simulink model "fourBusCase1"  (R2018b)
settings: Solver=FixedStepAuto  StartTime=0  StopTime=5  FixedStep=Ts  RelTol=1e-3
StartFcn:
  | clear
  | UserData = '4bus_case1.xlsx';
  | SimplusGT.Toolbox.Main();
undefined symbols (not defined in the file): ApparatusDiscreDamping, ApparatusPara, ApparatusPowerFlow, ApparatusType, OtherInputs, Ts, Wbase, x_e, Ybase, Zbase
libraries: powerlib x16, SimplusGT x7
settings Model: Creator=y_zhu  LastModifiedBy=y_zhu

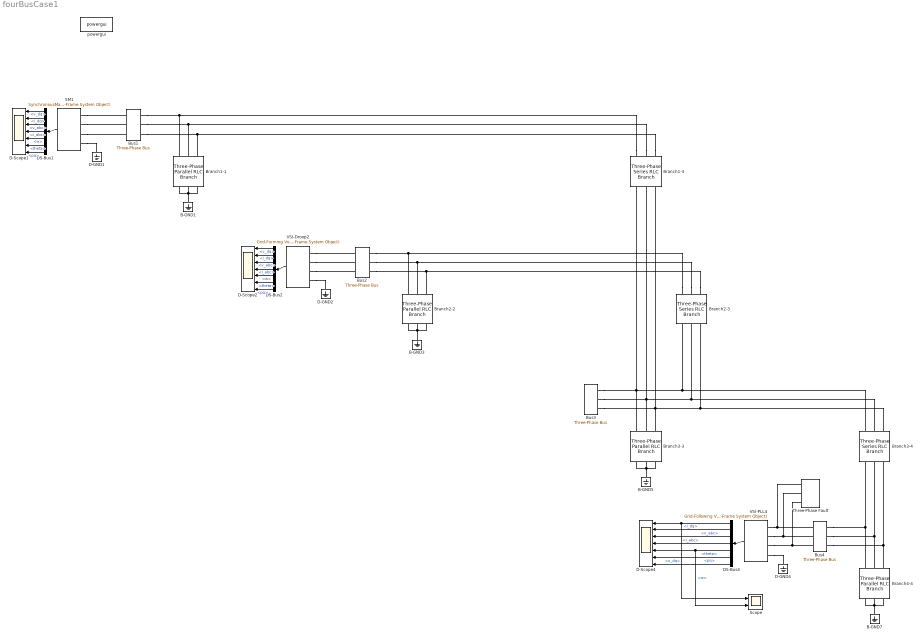
== system fourBusCase1 ==
  B-GND{1,3,5,7} (4 alike) : powerlib/Elements/Ground  LConnTagsString=a
  Branch1-1 : powerlib/Elements/Three-Phase Parallel RLC Branch  LConnTagsString=A|B|C  RConnTagsString=A|B|C  BranchType=RC  Resistance=(0.16534)*Zbase  Inductance=(Inf)*Zbase/Wbase  Capacitance=(0.238)*Ybase/Wbase  Measurements=None
      settings: SourceProductName=Simscape Power Systems  SourceProductBaseCode=PS
  Branch1-3 : powerlib/Elements/Three-Phase Series RLC Branch  LConnTagsString=A|B|C  RConnTagsString=A|B|C  BranchType=RL  Resistance=(0.004)*Zbase  Inductance=(0.057)*Zbase/Wbase  Capacitance=1e-6  Measurements=None
  Branch2-2 : powerlib/Elements/Three-Phase Parallel RLC Branch  LConnTagsString=A|B|C  RConnTagsString=A|B|C  BranchType=RLC  Resistance=(15.9719)*Zbase  Inductance=(41.1523)*Zbase/Wbase  Capacitance=(0.0368)*Ybase/Wbase  Measurements=None
      settings: SourceProductName=Simscape Power Systems  SourceProductBaseCode=PS
  Branch2-3 : powerlib/Elements/Three-Phase Series RLC Branch  LConnTagsString=A|B|C  RConnTagsString=A|B|C  BranchType=RL  Resistance=(0.0029)*Zbase  Inductance=(0.0734)*Zbase/Wbase  Capacitance=1e-6  Measurements=None
  Branch3-3 : powerlib/Elements/Three-Phase Parallel RLC Branch  LConnTagsString=A|B|C  RConnTagsString=A|B|C  BranchType=RLC  Resistance=(12.2146)*Zbase  Inductance=(12.216)*Zbase/Wbase  Capacitance=(2.142)*Ybase/Wbase  Measurements=None
      settings: SourceProductName=Simscape Power Systems  SourceProductBaseCode=PS
  Branch3-4 : powerlib/Elements/Three-Phase Series RLC Branch  LConnTagsString=A|B|C  RConnTagsString=A|B|C  BranchType=L  Resistance=(0)*Zbase  Inductance=(0.039)*Zbase/Wbase  Capacitance=1e-6  Measurements=None
  Branch4-4 : powerlib/Elements/Three-Phase Parallel RLC Branch  LConnTagsString=A|B|C  RConnTagsString=A|B|C  BranchType=RC  Resistance=(0.25293)*Zbase  Inductance=(Inf)*Zbase/Wbase  Capacitance=(0.95725)*Ybase/Wbase  Measurements=None
      settings: SourceProductName=Simscape Power Systems  SourceProductBaseCode=PS
  Bus{1..4} (4 alike) : SimplusGT/Three-Phase Bus  Vbase=1  Sbase=1
      settings: SourceProductName=Simplus Grid Tool
  D-GND1 : powerlib/Elements/Ground  LConnTagsString=a
  D-GND2 : powerlib/Elements/Ground  LConnTagsString=a
  D-GND4 : powerlib/Elements/Ground  LConnTagsString=a
  D-Scope1 : Scope  NumInputPorts=7
  D-Scope2 : Scope  NumInputPorts=7
  D-Scope4 : Scope  NumInputPorts=7
  DS-Bus1 : BusSelector  OutputSignals=v_dq,i_dq,v_abc,i_abc,w,theta,pq
  DS-Bus2 : BusSelector  OutputSignals=v_dq,i_dq,v_abc,i_abc,w,theta,pq
  DS-Bus4 : BusSelector  OutputSignals=v_dq,i_dq,v_abc,i_abc,w,theta,pq
  SM1 : SimplusGT/SynchronousMachineFull_Cyp_SMAVRPSSGOV (dq-Frame System Object)  Ts=Ts  Sbase=Sbase  Vbase=Vbase  Wbase=Wbase  ApparatusType=ApparatusType{1}  ApparatusPara=ApparatusPara{1}  PowerFlow=ApparatusPowerFlow{1}  x0=x_e{1}  OtherInputs=OtherInputs{1}  DiscreMethod=Hybrid Trapezoidal  EnableInsideModification=off  DiscreDampingFlag=on  DiscreDampingValue=ApparatusDiscreDamping{1}  LinearizationTimes=1  DirectFeedthrough=off
      settings: SourceProductName=Simplus Grid Tool
  Scope : Scope  NumInputPorts=2
  Three-Phase Fault : powerlib/Elements/Three-Phase Fault  InitialStates=0  FaultA=on  FaultB=on  FaultC=on  GroundFault=on  SwitchTimes="[2+1/60  2+3/60]"  External=off  SwitchStatus=NaN  FaultResistance=0.001  GroundResistance=0.01  SnubberResistance=1e6  SnubberCapacitance=inf  Measurements=None
  VSI-Droop2 : SimplusGT/Grid-Forming Voltage-Source Inverter (dq-Frame System Object)  Ts=Ts  Sbase=Sbase  Vbase=Vbase  Wbase=Wbase  ApparatusType=ApparatusType{2}  ApparatusPara=ApparatusPara{2}  PowerFlow=ApparatusPowerFlow{2}  x0=x_e{2}  OtherInputs=OtherInputs{2}  DiscreMethod=Hybrid Trapezoidal  EnableInsideModification=off  DiscreDampingFlag=on  DiscreDampingValue=ApparatusDiscreDamping{2}  LinearizationTimes=1  DirectFeedthrough=off
      settings: SourceProductName=Simplus Grid Tool
  VSI-PLL4 : SimplusGT/Grid-Following Voltage-Source Inverter (dq-Frame System Object)  Ts=Ts  Sbase=Sbase  Vbase=Vbase  Wbase=Wbase  ApparatusType=ApparatusType{4}  ApparatusPara=ApparatusPara{4}  PowerFlow=ApparatusPowerFlow{4}  x0=x_e{4}  OtherInputs=OtherInputs{4}  DiscreMethod=Hybrid Trapezoidal  EnableInsideModification=off  DiscreDampingFlag=on  DiscreDampingValue=ApparatusDiscreDamping{4}  LinearizationTimes=1  DirectFeedthrough=off
      settings: SourceProductName=Simplus Grid Tool
  powergui : powerlib/powergui  Priority=1  SimulationMode=Discrete  SampleTime=Ts  frequency=60  Iterations=50  frequencyindice=0  Pbase=100e6  ErrMax=1e-4  UnitsV=kV  UnitsW=MW  buscounter=0  FunctionMessages=off  echomessages=off  EnableUseOfTLC=off  CurrentSourceSwitches=off  DisableSnubberDevices=off  DisableRonSwitches=off  DisableVfSwitches=off  DisplayEquations=off  SolverType=Tustin/Backward Euler (TBE)  Interpol=off  ExternalGateDelay=off  methode=off  Ts=100  x0status=blocks  SPID=off  SwTol=0  HookPort=off  RestoreLinks=warning  ResistiveCurrentMeasurement=off  Frange=[0:2:500]  Ylog=off  Xlog=on  ShowGrid=off  save=off  variable=ZData  structure=0  ZoomFFT=off  StartTime=0.0  cycles=1  DisplayStyle=1  fundamental=60  FreqAxis=off  MaxFrequency=1000  frequencyindicesteady=1  RmsSteady=1  display=off
  wires:
  SM1/1 -> DS-Bus1/1
  DS-Bus1/1 -> D-Scope1/1  "<v_dq>"
  DS-Bus1/2 -> D-Scope1/2  "<i_dq>"
  DS-Bus1/3 -> D-Scope1/3  "<v_abc>"
  DS-Bus1/4 -> D-Scope1/4  "<i_abc>"
  DS-Bus1/5 -> D-Scope1/5  "<w>"
  DS-Bus1/6 -> D-Scope1/6  "<theta>"
  DS-Bus1/7 -> D-Scope1/7  "<pq>"
  VSI-Droop2/1 -> DS-Bus2/1
  DS-Bus2/1 -> D-Scope2/1  "<v_dq>"
  DS-Bus2/2 -> D-Scope2/2  "<i_dq>"
  DS-Bus2/3 -> D-Scope2/3  "<v_abc>"
  DS-Bus2/4 -> D-Scope2/4  "<i_abc>"
  DS-Bus2/5 -> D-Scope2/5  "<w>"
  DS-Bus2/6 -> D-Scope2/6  "<theta>"
  DS-Bus2/7 -> D-Scope2/7  "<pq>"
  VSI-PLL4/1 -> DS-Bus4/1
  DS-Bus4/2 -> D-Scope4/2  "<i_dq>"
  DS-Bus4/3 -> D-Scope4/3  "<v_abc>"
  DS-Bus4/5 -> Scope/2, D-Scope4/5  "<w>"
  DS-Bus4/6 -> D-Scope4/6  "<theta>"
  DS-Bus4/7 -> D-Scope4/7  "<pq>"
  DS-Bus4/1 -> Scope/1, D-Scope4/1  "<v_dq>"
  DS-Bus4/4 -> D-Scope4/4  "<i_abc>"
  connections:
  SM1/LConn4 -- D-GND1/LConn1
  VSI-Droop2/LConn4 -- D-GND2/LConn1
  VSI-PLL4/LConn4 -- D-GND4/LConn1
  Branch1-1/RConn1 -- Branch1-1/RConn2 -- Branch1-1/RConn3 -- B-GND1/LConn1
  Branch2-2/RConn1 -- Branch2-2/RConn2 -- Branch2-2/RConn3 -- B-GND3/LConn1
  Branch3-3/RConn1 -- Branch3-3/RConn2 -- Branch3-3/RConn3 -- B-GND5/LConn1
  Branch4-4/RConn1 -- Branch4-4/RConn2 -- Branch4-4/RConn3 -- B-GND7/LConn1
  Branch1-3/RConn1 -- Bus3/RConn1 -- Branch3-3/LConn1 -- Branch3-4/LConn1 -- Branch2-3/RConn1
  Branch1-3/RConn2 -- Bus3/RConn2 -- Branch3-3/LConn2 -- Branch3-4/LConn2 -- Branch2-3/RConn2
  Branch1-3/RConn3 -- Bus3/RConn3 -- Branch3-3/LConn3 -- Branch3-4/LConn3 -- Branch2-3/RConn3
  Branch1-3/LConn1 -- Bus1/RConn1 -- Branch1-1/LConn1
  Branch1-3/LConn2 -- Bus1/RConn2 -- Branch1-1/LConn2
  Branch1-3/LConn3 -- Bus1/RConn3 -- Branch1-1/LConn3
  Branch2-3/LConn1 -- Bus2/RConn1 -- Branch2-2/LConn1
  Branch2-3/LConn2 -- Bus2/RConn2 -- Branch2-2/LConn2
  Branch2-3/LConn3 -- Bus2/RConn3 -- Branch2-2/LConn3
  Branch3-4/RConn1 -- Bus4/RConn1 -- Branch4-4/LConn1
  Branch3-4/RConn2 -- Bus4/RConn2 -- Branch4-4/LConn2
  Branch3-4/RConn3 -- Bus4/RConn3 -- Branch4-4/LConn3
  SM1/LConn1 -- Bus1/LConn1
  SM1/LConn2 -- Bus1/LConn2
  SM1/LConn3 -- Bus1/LConn3
  VSI-Droop2/LConn1 -- Bus2/LConn1
  VSI-Droop2/LConn2 -- Bus2/LConn2
  VSI-Droop2/LConn3 -- Bus2/LConn3
  VSI-PLL4/LConn1 -- Three-Phase Fault/LConn1 -- Bus4/LConn1
  VSI-PLL4/LConn2 -- Three-Phase Fault/LConn2 -- Bus4/LConn2
  VSI-PLL4/LConn3 -- Three-Phase Fault/LConn3 -- Bus4/LConn3
